simulink model "single_port_bram_test"  (R2018a)
(part 2 of 56)

      mask prompts: io_names "Names [msb...lsb]"; io_widths "Bitwidths [msb...lsb]"; io_bps "Binary pts [msb...lsb]"; io_types "Data types [msb...lsb], ufix=0, fix=1, bool=2"; show_format "Print format string?"; snap_storage "Storage medium"; snap_dram_dimm "DRAM dimm"; snap_dram_clock "DRAM clock rate"; snap_nsamples "Number of Samples (2^?)"; snap_data_width "Data width"; snap_offset "Start delay support"; snap_circap "Circular capture support"; snap_value "Extra value capture support"; snap_ext_arm "External arm support"; snap_ext_circ "External circular capture support"; snap_provide_outputs "Provide outputs"; snap_use_dsp48 "Use DSP48s to implement counters"; snap_delay "Pre-snapshot delay"; extra_names "Names [msb...lsb]"; extra_widths "Widths [msb...lsb]"; extra_bps "Binary pts [msb...lsb]"; extra_types "Data types [msb...lsb], ufix=0, fix=1, bool=2"
      mask help:
      | A wrapped snapshot block. Allows specification of inputs to a snapblock word so the toolflow can automatically set up the scope.
      | See documentation for snapshot for explanation of parameters.
      mask init:
      | bitsnap_init(gcb);
      settings: AttributesFormatString=|
      | snap(5):uf8.0,uf8.0,b,b,b = 19 bits\n32 wide, 8192 deep
      | debugID: 63192898
      mask TypeOptions snap_storage: bram | dram
      mask Callback snap_storage: bitsnap_callback();
      mask TypeOptions snap_dram_dimm: 1 | 2 | 3 | 4
      mask TypeOptions snap_dram_clock: 200 | 250 | 266 | 300 | 333
      mask TypeOptions snap_data_width: 8 | 16 | 32 | 64 | 128
      mask Callback snap_value: bitsnap_callback();
      mask Callback snap_ext_arm: bitsnap_callback();
      mask Callback snap_ext_circ: bitsnap_callback();
      mask Callback snap_provide_outputs: bitsnap_callback();
      mask DialogControl ParameterTabVar0 Prompt: Inputs
      mask DialogControl ParameterTabVar01 Prompt: Snapshot
      mask DialogControl ParameterTabVar012 Prompt: Extra Value
  snap_cnt5 : Subsystem  Tag=casper:bitsnap  Commented=on  AncestorBlock=casper_library_scopes/bitfield_snapshot  mask(bitsnap){io_names=bram_in bram_out dv_in dv_out trig], io_widths=[8 8 1 1 1], io_bps=[0 0 0 0 0], io_types=[0 0 2 2 2], show_format=on, snap_storage=bram, snap_dram_dimm=2, snap_dram_clock=250, snap_nsamples=13, snap_data_width=32, snap_offset=off, snap_circap=off, snap_value=off, snap_ext_arm=off, snap_ext_circ=off, snap_provide_outputs=on, snap_use_dsp48=on, snap_delay=2, extra_names=[c d], extra_widths=[30 2], extra_bps=[0 0], extra_types=[0 0]}
      mask prompts: io_names "Names [msb...lsb]"; io_widths "Bitwidths [msb...lsb]"; io_bps "Binary pts [msb...lsb]"; io_types "Data types [msb...lsb], ufix=0, fix=1, bool=2"; show_format "Print format string?"; snap_storage "Storage medium"; snap_dram_dimm "DRAM dimm"; snap_dram_clock "DRAM clock rate"; snap_nsamples "Number of Samples (2^?)"; snap_data_width "Data width"; snap_offset "Start delay support"; snap_circap "Circular capture support"; snap_value "Extra value capture support"; snap_ext_arm "External arm support"; snap_ext_circ "External circular capture support"; snap_provide_outputs "Provide outputs"; snap_use_dsp48 "Use DSP48s to implement counters"; snap_delay "Pre-snapshot delay"; extra_names "Names [msb...lsb]"; extra_widths "Widths [msb...lsb]"; extra_bps "Binary pts [msb...lsb]"; extra_types "Data types [msb...lsb], ufix=0, fix=1, bool=2"
      mask help:
      | A wrapped snapshot block. Allows specification of inputs to a snapblock word so the toolflow can automatically set up the scope.
      | See documentation for snapshot for explanation of parameters.
      mask init:
      | bitsnap_init(gcb);
      settings: AttributesFormatString=|
      | snap(5):uf8.0,uf8.0,b,b,b = 19 bits\n32 wide, 8192 deep
      | debugID: 63222689
      mask TypeOptions snap_storage: bram | dram
      mask Callback snap_storage: bitsnap_callback();
      mask TypeOptions snap_dram_dimm: 1 | 2 | 3 | 4
      mask TypeOptions snap_dram_clock: 200 | 250 | 266 | 300 | 333
      mask TypeOptions snap_data_width: 8 | 16 | 32 | 64 | 128
      mask Callback snap_value: bitsnap_callback();
      mask Callback snap_ext_arm: bitsnap_callback();
      mask Callback snap_ext_circ: bitsnap_callback();
      mask Callback snap_provide_outputs: bitsnap_callback();
      mask DialogControl ParameterTabVar0 Prompt: Inputs
      mask DialogControl ParameterTabVar01 Prompt: Snapshot
      mask DialogControl ParameterTabVar012 Prompt: Extra Value
  snap_cnt6 : Subsystem  Tag=casper:bitsnap  Commented=on  AncestorBlock=casper_library_scopes/bitfield_snapshot  mask(bitsnap){io_names=bram_in bram_out dv_in dv_out trig], io_widths=[8 8 1 1 1], io_bps=[0 0 0 0 0], io_types=[0 0 2 2 2], show_format=on, snap_storage=bram, snap_dram_dimm=2, snap_dram_clock=250, snap_nsamples=13, snap_data_width=32, snap_offset=off, snap_circap=off, snap_value=off, snap_ext_arm=off, snap_ext_circ=off, snap_provide_outputs=on, snap_use_dsp48=on, snap_delay=2, extra_names=[c d], extra_widths=[30 2], extra_bps=[0 0], extra_types=[0 0]}
      mask prompts: io_names "Names [msb...lsb]"; io_widths "Bitwidths [msb...lsb]"; io_bps "Binary pts [msb...lsb]"; io_types "Data types [msb...lsb], ufix=0, fix=1, bool=2"; show_format "Print format string?"; snap_storage "Storage medium"; snap_dram_dimm "DRAM dimm"; snap_dram_clock "DRAM clock rate"; snap_nsamples "Number of Samples (2^?)"; snap_data_width "Data width"; snap_offset "Start delay support"; snap_circap "Circular capture support"; snap_value "Extra value capture support"; snap_ext_arm "External arm support"; snap_ext_circ "External circular capture support"; snap_provide_outputs "Provide outputs"; snap_use_dsp48 "Use DSP48s to implement counters"; snap_delay "Pre-snapshot delay"; extra_names "Names [msb...lsb]"; extra_widths "Widths [msb...lsb]"; extra_bps "Binary pts [msb...lsb]"; extra_types "Data types [msb...lsb], ufix=0, fix=1, bool=2"
      mask help:
      | A wrapped snapshot block. Allows specification of inputs to a snapblock word so the toolflow can automatically set up the scope.
      | See documentation for snapshot for explanation of parameters.
      mask init:
      | bitsnap_init(gcb);
      settings: AttributesFormatString=|
      | snap(5):uf8.0,uf8.0,b,b,b = 19 bits\n32 wide, 8192 deep
      | debugID: 63252480
      mask TypeOptions snap_storage: bram | dram
      mask Callback snap_storage: bitsnap_callback();
      mask TypeOptions snap_dram_dimm: 1 | 2 | 3 | 4
      mask TypeOptions snap_dram_clock: 200 | 250 | 266 | 300 | 333
      mask TypeOptions snap_data_width: 8 | 16 | 32 | 64 | 128
      mask Callback snap_value: bitsnap_callback();
      mask Callback snap_ext_arm: bitsnap_callback();
      mask Callback snap_ext_circ: bitsnap_callback();
      mask Callback snap_provide_outputs: bitsnap_callback();
      mask DialogControl ParameterTabVar0 Prompt: Inputs
      mask DialogControl ParameterTabVar01 Prompt: Snapshot
      mask DialogControl ParameterTabVar012 Prompt: Extra Value
  snap_cnt7 : Subsystem  Tag=casper:bitsnap  Commented=on  AncestorBlock=casper_library_scopes/bitfield_snapshot  mask(bitsnap){io_names=bram_in bram_out dv_in dv_out trig], io_widths=[8 8 1 1 1], io_bps=[0 0 0 0 0], io_types=[0 0 2 2 2], show_format=on, snap_storage=bram, snap_dram_dimm=2, snap_dram_clock=250, snap_nsamples=13, snap_data_width=32, snap_offset=off, snap_circap=off, snap_value=off, snap_ext_arm=off, snap_ext_circ=off, snap_provide_outputs=on, snap_use_dsp48=on, snap_delay=2, extra_names=[c d], extra_widths=[30 2], extra_bps=[0 0], extra_types=[0 0]}
      mask prompts: io_names "Names [msb...lsb]"; io_widths "Bitwidths [msb...lsb]"; io_bps "Binary pts [msb...lsb]"; io_types "Data types [msb...lsb], ufix=0, fix=1, bool=2"; show_format "Print format string?"; snap_storage "Storage medium"; snap_dram_dimm "DRAM dimm"; snap_dram_clock "DRAM clock rate"; snap_nsamples "Number of Samples (2^?)"; snap_data_width "Data width"; snap_offset "Start delay support"; snap_circap "Circular capture support"; snap_value "Extra value capture support"; snap_ext_arm "External arm support"; snap_ext_circ "External circular capture support"; snap_provide_outputs "Provide outputs"; snap_use_dsp48 "Use DSP48s to implement counters"; snap_delay "Pre-snapshot delay"; extra_names "Names [msb...lsb]"; extra_widths "Widths [msb...lsb]"; extra_bps "Binary pts [msb...lsb]"; extra_types "Data types [msb...lsb], ufix=0, fix=1, bool=2"
      mask help:
      | A wrapped snapshot block. Allows specification of inputs to a snapblock word so the toolflow can automatically set up the scope.
      | See documentation for snapshot for explanation of parameters.
      mask init:
      | bitsnap_init(gcb);
      settings: AttributesFormatString=|
      | snap(5):uf8.0,uf8.0,b,b,b = 19 bits\n32 wide, 8192 deep
      | debugID: 63282271
      mask TypeOptions snap_storage: bram | dram
      mask Callback snap_storage: bitsnap_callback();
      mask TypeOptions snap_dram_dimm: 1 | 2 | 3 | 4
      mask TypeOptions snap_dram_clock: 200 | 250 | 266 | 300 | 333
      mask TypeOptions snap_data_width: 8 | 16 | 32 | 64 | 128
      mask Callback snap_value: bitsnap_callback();
      mask Callback snap_ext_arm: bitsnap_callback();
      mask Callback snap_ext_circ: bitsnap_callback();
      mask Callback snap_provide_outputs: bitsnap_callback();
      mask DialogControl ParameterTabVar0 Prompt: Inputs
      mask DialogControl ParameterTabVar01 Prompt: Snapshot
      mask DialogControl ParameterTabVar012 Prompt: Extra Value
  snap_dp1 : Subsystem  Tag=casper:bitsnap  Commented=on  AncestorBlock=casper_library_scopes/bitfield_snapshot  mask(bitsnap){io_names=bram_in bram_out dv_in dv_out trig], io_widths=[8 8 1 1 1], io_bps=[0 0 0 0 0], io_types=[0 0 2 2 2], show_format=on, snap_storage=bram, snap_dram_dimm=2, snap_dram_clock=250, snap_nsamples=13, snap_data_width=32, snap_offset=off, snap_circap=off, snap_value=off, snap_ext_arm=off, snap_ext_circ=off, snap_provide_outputs=on, snap_use_dsp48=on, snap_delay=2, extra_names=[c d], extra_widths=[30 2], extra_bps=[0 0], extra_types=[0 0]}
      mask prompts: io_names "Names [msb...lsb]"; io_widths "Bitwidths [msb...lsb]"; io_bps "Binary pts [msb...lsb]"; io_types "Data types [msb...lsb], ufix=0, fix=1, bool=2"; show_format "Print format string?"; snap_storage "Storage medium"; snap_dram_dimm "DRAM dimm"; snap_dram_clock "DRAM clock rate"; snap_nsamples "Number of Samples (2^?)"; snap_data_width "Data width"; snap_offset "Start delay support"; snap_circap "Circular capture support"; snap_value "Extra value capture support"; snap_ext_arm "External arm support"; snap_ext_circ "External circular capture support"; snap_provide_outputs "Provide outputs"; snap_use_dsp48 "Use DSP48s to implement counters"; snap_delay "Pre-snapshot delay"; extra_names "Names [msb...lsb]"; extra_widths "Widths [msb...lsb]"; extra_bps "Binary pts [msb...lsb]"; extra_types "Data types [msb...lsb], ufix=0, fix=1, bool=2"
      mask help:
      | A wrapped snapshot block. Allows specification of inputs to a snapblock word so the toolflow can automatically set up the scope.
      | See documentation for snapshot for explanation of parameters.
      mask init:
      | bitsnap_init(gcb);
      settings: AttributesFormatString=|
      | snap(5):uf8.0,uf8.0,b,b,b = 19 bits\n32 wide, 8192 deep
      | debugID: 34845580
      mask TypeOptions snap_storage: bram | dram
      mask Callback snap_storage: bitsnap_callback();
      mask TypeOptions snap_dram_dimm: 1 | 2 | 3 | 4
      mask TypeOptions snap_dram_clock: 200 | 250 | 266 | 300 | 333
      mask TypeOptions snap_data_width: 8 | 16 | 32 | 64 | 128
      mask Callback snap_value: bitsnap_callback();
      mask Callback snap_ext_arm: bitsnap_callback();
      mask Callback snap_ext_circ: bitsnap_callback();
      mask Callback snap_provide_outputs: bitsnap_callback();
      mask DialogControl ParameterTabVar0 Prompt: Inputs
      mask DialogControl ParameterTabVar01 Prompt: Snapshot
      mask DialogControl ParameterTabVar012 Prompt: Extra Value
  snap_dp2 : Subsystem  Tag=casper:bitsnap  Commented=on  AncestorBlock=casper_library_scopes/bitfield_snapshot  mask(bitsnap){io_names=bram_in bram_out dv_in dv_out trig], io_widths=[8 8 1 1 1], io_bps=[0 0 0 0 0], io_types=[0 0 2 2 2], show_format=on, snap_storage=bram, snap_dram_dimm=2, snap_dram_clock=250, snap_nsamples=13, snap_data_width=32, snap_offset=off, snap_circap=off, snap_value=off, snap_ext_arm=off, snap_ext_circ=off, snap_provide_outputs=on, snap_use_dsp48=on, snap_delay=2, extra_names=[c d], extra_widths=[30 2], extra_bps=[0 0], extra_types=[0 0]}
      mask prompts: io_names "Names [msb...lsb]"; io_widths "Bitwidths [msb...lsb]"; io_bps "Binary pts [msb...lsb]"; io_types "Data types [msb...lsb], ufix=0, fix=1, bool=2"; show_format "Print format string?"; snap_storage "Storage medium"; snap_dram_dimm "DRAM dimm"; snap_dram_clock "DRAM clock rate"; snap_nsamples "Number of Samples (2^?)"; snap_data_width "Data width"; snap_offset "Start delay support"; snap_circap "Circular capture support"; snap_value "Extra value capture support"; snap_ext_arm "External arm support"; snap_ext_circ "External circular capture support"; snap_provide_outputs "Provide outputs"; snap_use_dsp48 "Use DSP48s to implement counters"; snap_delay "Pre-snapshot delay"; extra_names "Names [msb...lsb]"; extra_widths "Widths [msb...lsb]"; extra_bps "Binary pts [msb...lsb]"; extra_types "Data types [msb...lsb], ufix=0, fix=1, bool=2"
      mask help:
      | A wrapped snapshot block. Allows specification of inputs to a snapblock word so the toolflow can automatically set up the scope.
      | See documentation for snapshot for explanation of parameters.
      mask init:
      | bitsnap_init(gcb);
      settings: AttributesFormatString=|
      | snap(5):uf8.0,uf8.0,b,b,b = 19 bits\n32 wide, 8192 deep
      | debugID: 34875371
      mask TypeOptions snap_storage: bram | dram
      mask Callback snap_storage: bitsnap_callback();
      mask TypeOptions snap_dram_dimm: 1 | 2 | 3 | 4
      mask TypeOptions snap_dram_clock: 200 | 250 | 266 | 300 | 333
      mask TypeOptions snap_data_width: 8 | 16 | 32 | 64 | 128
      mask Callback snap_value: bitsnap_callback();
      mask Callback snap_ext_arm: bitsnap_callback();
      mask Callback snap_ext_circ: bitsnap_callback();
      mask Callback snap_provide_outputs: bitsnap_callback();
      mask DialogControl ParameterTabVar0 Prompt: Inputs
      mask DialogControl ParameterTabVar01 Prompt: Snapshot
      mask DialogControl ParameterTabVar012 Prompt: Extra Value
  snap_dp3 : Subsystem  Tag=casper:bitsnap  Commented=on  AncestorBlock=casper_library_scopes/bitfield_snapshot  mask(bitsnap){io_names=bram_in bram_out dv_in dv_out trig], io_widths=[8 8 1 1 1], io_bps=[0 0 0 0 0], io_types=[0 0 2 2 2], show_format=on, snap_storage=bram, snap_dram_dimm=2, snap_dram_clock=250, snap_nsamples=13, snap_data_width=32, snap_offset=off, snap_circap=off, snap_value=off, snap_ext_arm=off, snap_ext_circ=off, snap_provide_outputs=on, snap_use_dsp48=on, snap_delay=2, extra_names=[c d], extra_widths=[30 2], extra_bps=[0 0], extra_types=[0 0]}
      mask prompts: io_names "Names [msb...lsb]"; io_widths "Bitwidths [msb...lsb]"; io_bps "Binary pts [msb...lsb]"; io_types "Data types [msb...lsb], ufix=0, fix=1, bool=2"; show_format "Print format string?"; snap_storage "Storage medium"; snap_dram_dimm "DRAM dimm"; snap_dram_clock "DRAM clock rate"; snap_nsamples "Number of Samples (2^?)"; snap_data_width "Data width"; snap_offset "Start delay support"; snap_circap "Circular capture support"; snap_value "Extra value capture support"; snap_ext_arm "External arm support"; snap_ext_circ "External circular capture support"; snap_provide_outputs "Provide outputs"; snap_use_dsp48 "Use DSP48s to implement counters"; snap_delay "Pre-snapshot delay"; extra_names "Names [msb...lsb]"; extra_widths "Widths [msb...lsb]"; extra_bps "Binary pts [msb...lsb]"; extra_types "Data types [msb...lsb], ufix=0, fix=1, bool=2"
      mask help:
      | A wrapped snapshot block. Allows specification of inputs to a snapblock word so the toolflow can automatically set up the scope.
      | See documentation for snapshot for explanation of parameters.
      mask init:
      | bitsnap_init(gcb);
      settings: AttributesFormatString=|
      | snap(5):uf8.0,uf8.0,b,b,b = 19 bits\n32 wide, 8192 deep
      | debugID: 34905162
      mask TypeOptions snap_storage: bram | dram
      mask Callback snap_storage: bitsnap_callback();
      mask TypeOptions snap_dram_dimm: 1 | 2 | 3 | 4
      mask TypeOptions snap_dram_clock: 200 | 250 | 266 | 300 | 333
      mask TypeOptions snap_data_width: 8 | 16 | 32 | 64 | 128
      mask Callback snap_value: bitsnap_callback();
      mask Callback snap_ext_arm: bitsnap_callback();
      mask Callback snap_ext_circ: bitsnap_callback();
      mask Callback snap_provide_outputs: bitsnap_callback();
      mask DialogControl ParameterTabVar0 Prompt: Inputs
      mask DialogControl ParameterTabVar01 Prompt: Snapshot
      mask DialogControl ParameterTabVar012 Prompt: Extra Value
  snap_dp4 : Subsystem  Tag=casper:bitsnap  Commented=on  AncestorBlock=casper_library_scopes/bitfield_snapshot  mask(bitsnap){io_names=bram_in bram_out dv_in dv_out trig], io_widths=[8 8 1 1 1], io_bps=[0 0 0 0 0], io_types=[0 0 2 2 2], show_format=on, snap_storage=bram, snap_dram_dimm=2, snap_dram_clock=250, snap_nsamples=13, snap_data_width=32, snap_offset=off, snap_circap=off, snap_value=off, snap_ext_arm=off, snap_ext_circ=off, snap_provide_outputs=on, snap_use_dsp48=on, snap_delay=2, extra_names=[c d], extra_widths=[30 2], extra_bps=[0 0], extra_types=[0 0]}
      mask prompts: io_names "Names [msb...lsb]"; io_widths "Bitwidths [msb...lsb]"; io_bps "Binary pts [msb...lsb]"; io_types "Data types [msb...lsb], ufix=0, fix=1, bool=2"; show_format "Print format string?"; snap_storage "Storage medium"; snap_dram_dimm "DRAM dimm"; snap_dram_clock "DRAM clock rate"; snap_nsamples "Number of Samples (2^?)"; snap_data_width "Data width"; snap_offset "Start delay support"; snap_circap "Circular capture support"; snap_value "Extra value capture support"; snap_ext_arm "External arm support"; snap_ext_circ "External circular capture support"; snap_provide_outputs "Provide outputs"; snap_use_dsp48 "Use DSP48s to implement counters"; snap_delay "Pre-snapshot delay"; extra_names "Names [msb...lsb]"; extra_widths "Widths [msb...lsb]"; extra_bps "Binary pts [msb...lsb]"; extra_types "Data types [msb...lsb], ufix=0, fix=1, bool=2"
      mask help:
      | A wrapped snapshot block. Allows specification of inputs to a snapblock word so the toolflow can automatically set up the scope.
      | See documentation for snapshot for explanation of parameters.
      mask init:
      | bitsnap_init(gcb);
      settings: AttributesFormatString=|
      | snap(5):uf8.0,uf8.0,b,b,b = 19 bits\n32 wide, 8192 deep
      | debugID: 34934953
      mask TypeOptions snap_storage: bram | dram
      mask Callback snap_storage: bitsnap_callback();
      mask TypeOptions snap_dram_dimm: 1 | 2 | 3 | 4
      mask TypeOptions snap_dram_clock: 200 | 250 | 266 | 300 | 333
      mask TypeOptions snap_data_width: 8 | 16 | 32 | 64 | 128
      mask Callback snap_value: bitsnap_callback();
      mask Callback snap_ext_arm: bitsnap_callback();
      mask Callback snap_ext_circ: bitsnap_callback();
      mask Callback snap_provide_outputs: bitsnap_callback();
      mask DialogControl ParameterTabVar0 Prompt: Inputs
      mask DialogControl ParameterTabVar01 Prompt: Snapshot
      mask DialogControl ParameterTabVar012 Prompt: Extra Value
  snap_dp5 : Subsystem  Tag=casper:bitsnap  Commented=on  AncestorBlock=casper_library_scopes/bitfield_snapshot  mask(bitsnap){io_names=bram_in bram_out dv_in dv_out trig], io_widths=[8 8 1 1 1], io_bps=[0 0 0 0 0], io_types=[0 0 2 2 2], show_format=on, snap_storage=bram, snap_dram_dimm=2, snap_dram_clock=250, snap_nsamples=13, snap_data_width=32, snap_offset=off, snap_circap=off, snap_value=off, snap_ext_arm=off, snap_ext_circ=off, snap_provide_outputs=on, snap_use_dsp48=on, snap_delay=2, extra_names=[c d], extra_widths=[30 2], extra_bps=[0 0], extra_types=[0 0]}
      mask prompts: io_names "Names [msb...lsb]"; io_widths "Bitwidths [msb...lsb]"; io_bps "Binary pts [msb...lsb]"; io_types "Data types [msb...lsb], ufix=0, fix=1, bool=2"; show_format "Print format string?"; snap_storage "Storage medium"; snap_dram_dimm "DRAM dimm"; snap_dram_clock "DRAM clock rate"; snap_nsamples "Number of Samples (2^?)"; snap_data_width "Data width"; snap_offset "Start delay support"; snap_circap "Circular capture support"; snap_value "Extra value capture support"; snap_ext_arm "External arm support"; snap_ext_circ "External circular capture support"; snap_provide_outputs "Provide outputs"; snap_use_dsp48 "Use DSP48s to implement counters"; snap_delay "Pre-snapshot delay"; extra_names "Names [msb...lsb]"; extra_widths "Widths [msb...lsb]"; extra_bps "Binary pts [msb...lsb]"; extra_types "Data types [msb...lsb], ufix=0, fix=1, bool=2"
      mask help:
      | A wrapped snapshot block. Allows specification of inputs to a snapblock word so the toolflow can automatically set up the scope.
      | See documentation for snapshot for explanation of parameters.
      mask init:
      | bitsnap_init(gcb);
      settings: AttributesFormatString=|
      | snap(5):uf8.0,uf8.0,b,b,b = 19 bits\n32 wide, 8192 deep
      | debugID: 34964744
      mask TypeOptions snap_storage: bram | dram
      mask Callback snap_storage: bitsnap_callback();
      mask TypeOptions snap_dram_dimm: 1 | 2 | 3 | 4
      mask TypeOptions snap_dram_clock: 200 | 250 | 266 | 300 | 333
      mask TypeOptions snap_data_width: 8 | 16 | 32 | 64 | 128
      mask Callback snap_value: bitsnap_callback();
      mask Callback snap_ext_arm: bitsnap_callback();
      mask Callback snap_ext_circ: bitsnap_callback();
      mask Callback snap_provide_outputs: bitsnap_callback();
      mask DialogControl ParameterTabVar0 Prompt: Inputs
      mask DialogControl ParameterTabVar01 Prompt: Snapshot
      mask DialogControl ParameterTabVar012 Prompt: Extra Value
  snap_dp6 : Subsystem  Tag=casper:bitsnap  Commented=on  AncestorBlock=casper_library_scopes/bitfield_snapshot  mask(bitsnap){io_names=bram_in bram_out dv_in dv_out trig], io_widths=[8 8 1 1 1], io_bps=[0 0 0 0 0], io_types=[0 0 2 2 2], show_format=on, snap_storage=bram, snap_dram_dimm=2, snap_dram_clock=250, snap_nsamples=13, snap_data_width=32, snap_offset=off, snap_circap=off, snap_value=off, snap_ext_arm=off, snap_ext_circ=off, snap_provide_outputs=on, snap_use_dsp48=on, snap_delay=2, extra_names=[c d], extra_widths=[30 2], extra_bps=[0 0], extra_types=[0 0]}
      mask prompts: io_names "Names [msb...lsb]"; io_widths "Bitwidths [msb...lsb]"; io_bps "Binary pts [msb...lsb]"; io_types "Data types [msb...lsb], ufix=0, fix=1, bool=2"; show_format "Print format string?"; snap_storage "Storage medium"; snap_dram_dimm "DRAM dimm"; snap_dram_clock "DRAM clock rate"; snap_nsamples "Number of Samples (2^?)"; snap_data_width "Data width"; snap_offset "Start delay support"; snap_circap "Circular capture support"; snap_value "Extra value capture support"; snap_ext_arm "External arm support"; snap_ext_circ "External circular capture support"; snap_provide_outputs "Provide outputs"; snap_use_dsp48 "Use DSP48s to implement counters"; snap_delay "Pre-snapshot delay"; extra_names "Names [msb...lsb]"; extra_widths "Widths [msb...lsb]"; extra_bps "Binary pts [msb...lsb]"; extra_types "Data types [msb...lsb], ufix=0, fix=1, bool=2"
      mask help:
      | A wrapped snapshot block. Allows specification of inputs to a snapblock word so the toolflow can automatically set up the scope.
      | See documentation for snapshot for explanation of parameters.
      mask init:
      | bitsnap_init(gcb);
      settings: AttributesFormatString=|
      | snap(5):uf8.0,uf8.0,b,b,b = 19 bits\n32 wide, 8192 deep
      | debugID: 34994535
      mask TypeOptions snap_storage: bram | dram
      mask Callback snap_storage: bitsnap_callback();
      mask TypeOptions snap_dram_dimm: 1 | 2 | 3 | 4
      mask TypeOptions snap_dram_clock: 200 | 250 | 266 | 300 | 333
      mask TypeOptions snap_data_width: 8 | 16 | 32 | 64 | 128
      mask Callback snap_value: bitsnap_callback();
      mask Callback snap_ext_arm: bitsnap_callback();
      mask Callback snap_ext_circ: bitsnap_callback();
      mask Callback snap_provide_outputs: bitsnap_callback();
      mask DialogControl ParameterTabVar0 Prompt: Inputs
      mask DialogControl ParameterTabVar01 Prompt: Snapshot
      mask DialogControl ParameterTabVar012 Prompt: Extra Value
  snap_dp7 : Subsystem  Tag=casper:bitsnap  Commented=on  AncestorBlock=casper_library_scopes/bitfield_snapshot  mask(bitsnap){io_names=bram_in bram_out dv_in dv_out trig], io_widths=[8 8 1 1 1], io_bps=[0 0 0 0 0], io_types=[0 0 2 2 2], show_format=on, snap_storage=bram, snap_dram_dimm=2, snap_dram_clock=250, snap_nsamples=13, snap_data_width=32, snap_offset=off, snap_circap=off, snap_value=off, snap_ext_arm=off, snap_ext_circ=off, snap_provide_outputs=on, snap_use_dsp48=on, snap_delay=2, extra_names=[c d], extra_widths=[30 2], extra_bps=[0 0], extra_types=[0 0]}
      mask prompts: io_names "Names [msb...lsb]"; io_widths "Bitwidths [msb...lsb]"; io_bps "Binary pts [msb...lsb]"; io_types "Data types [msb...lsb], ufix=0, fix=1, bool=2"; show_format "Print format string?"; snap_storage "Storage medium"; snap_dram_dimm "DRAM dimm"; snap_dram_clock "DRAM clock rate"; snap_nsamples "Number of Samples (2^?)"; snap_data_width "Data width"; snap_offset "Start delay support"; snap_circap "Circular capture support"; snap_value "Extra value capture support"; snap_ext_arm "External arm support"; snap_ext_circ "External circular capture support"; snap_provide_outputs "Provide outputs"; snap_use_dsp48 "Use DSP48s to implement counters"; snap_delay "Pre-snapshot delay"; extra_names "Names [msb...lsb]"; extra_widths "Widths [msb...lsb]"; extra_bps "Binary pts [msb...lsb]"; extra_types "Data types [msb...lsb], ufix=0, fix=1, bool=2"
      mask help:
      | A wrapped snapshot block. Allows specification of inputs to a snapblock word so the toolflow can automatically set up the scope.
      | See documentation for snapshot for explanation of parameters.
      mask init:
      | bitsnap_init(gcb);
      settings: AttributesFormatString=|
      | snap(5):uf8.0,uf8.0,b,b,b = 19 bits\n32 wide, 8192 deep
      | debugID: 35024326
      mask TypeOptions snap_storage: bram | dram
      mask Callback snap_storage: bitsnap_callback();
      mask TypeOptions snap_dram_dimm: 1 | 2 | 3 | 4
      mask TypeOptions snap_dram_clock: 200 | 250 | 266 | 300 | 333
      mask TypeOptions snap_data_width: 8 | 16 | 32 | 64 | 128
      mask Callback snap_value: bitsnap_callback();
      mask Callback snap_ext_arm: bitsnap_callback();
      mask Callback snap_ext_circ: bitsnap_callback();
      mask Callback snap_provide_outputs: bitsnap_callback();
      mask DialogControl ParameterTabVar0 Prompt: Inputs
      mask DialogControl ParameterTabVar01 Prompt: Snapshot
      mask DialogControl ParameterTabVar012 Prompt: Extra Value
  snap_dp8 : Subsystem  Tag=casper:bitsnap  Commented=on  AncestorBlock=casper_library_scopes/bitfield_snapshot  mask(bitsnap){io_names=bram_in bram_out dv_in dv_out trig], io_widths=[8 8 1 1 1], io_bps=[0 0 0 0 0], io_types=[0 0 2 2 2], show_format=on, snap_storage=bram, snap_dram_dimm=2, snap_dram_clock=250, snap_nsamples=13, snap_data_width=32, snap_offset=off, snap_circap=off, snap_value=off, snap_ext_arm=off, snap_ext_circ=off, snap_provide_outputs=on, snap_use_dsp48=on, snap_delay=2, extra_names=[c d], extra_widths=[30 2], extra_bps=[0 0], extra_types=[0 0]}
      mask prompts: io_names "Names [msb...lsb]"; io_widths "Bitwidths [msb...lsb]"; io_bps "Binary pts [msb...lsb]"; io_types "Data types [msb...lsb], ufix=0, fix=1, bool=2"; show_format "Print format string?"; snap_storage "Storage medium"; snap_dram_dimm "DRAM dimm"; snap_dram_clock "DRAM clock rate"; snap_nsamples "Number of Samples (2^?)"; snap_data_width "Data width"; snap_offset "Start delay support"; snap_circap "Circular capture support"; snap_value "Extra value capture support"; snap_ext_arm "External arm support"; snap_ext_circ "External circular capture support"; snap_provide_outputs "Provide outputs"; snap_use_dsp48 "Use DSP48s to implement counters"; snap_delay "Pre-snapshot delay"; extra_names "Names [msb...lsb]"; extra_widths "Widths [msb...lsb]"; extra_bps "Binary pts [msb...lsb]"; extra_types "Data types [msb...lsb], ufix=0, fix=1, bool=2"
      mask help:
      | A wrapped snapshot block. Allows specification of inputs to a snapblock word so the toolflow can automatically set up the scope.
      | See documentation for snapshot for explanation of parameters.
      mask init:
      | bitsnap_init(gcb);
      settings: AttributesFormatString=|
      | snap(5):uf8.0,uf8.0,b,b,b = 19 bits\n32 wide, 8192 deep
      | debugID: 35054117
      mask TypeOptions snap_storage: bram | dram
      mask Callback snap_storage: bitsnap_callback();
      mask TypeOptions snap_dram_dimm: 1 | 2 | 3 | 4
      mask TypeOptions snap_dram_clock: 200 | 250 | 266 | 300 | 333
      mask TypeOptions snap_data_width: 8 | 16 | 32 | 64 | 128
      mask Callback snap_value: bitsnap_callback();
      mask Callback snap_ext_arm: bitsnap_callback();
      mask Callback snap_ext_circ: bitsnap_callback();
      mask Callback snap_provide_outputs: bitsnap_callback();
      mask DialogControl ParameterTabVar0 Prompt: Inputs
      mask DialogControl ParameterTabVar01 Prompt: Snapshot
      mask DialogControl ParameterTabVar012 Prompt: Extra Value
  sys_rst : Subsystem  Tag=xps:sw_reg  AncestorBlock=xps_library/Memory/software_register  mask(swreg){io_dir=From Processor, io_delay=1, init_val=0, sample_period=1, names=rst, bitwidths=1, bin_pts=0, arith_types=2, sim_port=on, show_format=on}
      mask prompts: io_dir "I/O direction"; io_delay "I/O delay"; init_val "Initial Value"; sample_period "Sample period"; names "Bitfield names [msb...lsb]"; bitwidths "Bitfield widths"; bin_pts "Bitfield binary pts"; arith_types "Bitfield types, ufix=0, fix=1, bool=2"; sim_port "Provide sim input/output?"; show_format "Print format string?"
      mask help: A 32-bit software-accessible register. Can be divided into bitfields of varying widths and types using the fields in the block mask.
      mask init:
      | swreg_init(gcb)
      settings: AttributesFormatString=1input:b = 1 bits
      mask TypeOptions io_dir: To Processor | From Processor
      mask Callback io_dir:
      | mask_enables = get_param(gcb, 'MaskEnables');
      | mask_names = get_param(gcb, 'MaskNames');
      | if strcmp(get_param(gcb, 'io_dir'), 'To Processor'),
      |     mask_enables{ismember(mask_names, 'sample_period')} = 'off';
      | else
      |     mask_enables{ismember(mask_names, 'sample_period')} = 'on';
      | end
      | set_param(gcb, 'MaskEnables', mask_enables);
      mask DialogControl ParameterTabVar0 Prompt: Setup
  sys_start : Subsystem  Tag=xps:sw_reg  AncestorBlock=xps_library/Memory/software_register  mask(swreg){io_dir=From Processor, io_delay=1, init_val=0, sample_period=1, names=en, bitwidths=1, bin_pts=0, arith_types=2, sim_port=on, show_format=on}
      mask prompts: io_dir "I/O direction"; io_delay "I/O delay"; init_val "Initial Value"; sample_period "Sample period"; names "Bitfield names [msb...lsb]"; bitwidths "Bitfield widths"; bin_pts "Bitfield binary pts"; arith_types "Bitfield types, ufix=0, fix=1, bool=2"; sim_port "Provide sim input/output?"; show_format "Print format string?"
      mask help: A 32-bit software-accessible register. Can be divided into bitfields of varying widths and types using the fields in the block mask.
      mask init:
      | swreg_init(gcb)
      settings: AttributesFormatString=1input:b = 1 bits
      mask TypeOptions io_dir: To Processor | From Processor
      mask Callback io_dir:
      | mask_enables = get_param(gcb, 'MaskEnables');
      | mask_names = get_param(gcb, 'MaskNames');
      | if strcmp(get_param(gcb, 'io_dir'), 'To Processor'),
      |     mask_enables{ismember(mask_names, 'sample_period')} = 'off';
      | else
      |     mask_enables{ismember(mask_names, 'sample_period')} = 'on';
      | end
      | set_param(gcb, 'MaskEnables', mask_enables);
      mask DialogControl ParameterTabVar0 Prompt: Setup
  xsg_core_config : xps_library/Platforms/SKARAB  Tag=xps:xsg  hw_sys=SKARAB:xc7vx690t  clk_src=sys_clk  clk_rate=238  sample_period=1  synthesis_tool=XST
      settings: SourceProductName=CASPER XPS Blockset
  wires:
  ram/1 -> Gateway Out5/1, pipeline3/1(d)
  pipeline112/1(q) -> [forty_gbe_rx_eof]
  Constant23/1 -> [s256_v]
  Logical7/1 -> Logical5/1
  [board_in_fault] -> Inverter/1
  [force_gbe_txen] -> Logical7/2
  pipeline97/1(q) -> gbe0/4(tx_dest_ip)
  pipeline62/1(q) -> [forty_gbe_rx_valid]
  Logical2/1 -> gbe0/3(tx_valid)
  [s256_eof] -> Delay4/2
  pipeline114/1(q) -> [forty_gbe_rx_overrun]
  gbe0/1(led_up) -> pipeline100/1(d)
  pipeline108/1(q) -> [forty_gbe_rx_data]
  pipeline102/1(q) -> [forty_gbe_led_tx]
  Constant22/1 -> [s256_d]
  pipeline104/1(q) -> [forty_gbe_tx_of]
  pipeline22/1(q) -> gbe_status/2(out_led_rx)
  pipeline103/1(q) -> [forty_gbe_tx_full]
  Logical5/1 -> Delay4/1
  pipeline99/1(q) -> gbe0/1(rst)
  [s256_eof] -> Logical3/2
  pipeline20/1(q) -> gbe_status/1(out_led_up)
  Constant7/1 -> [force_gbe_txen], [gbe_txen]
  gbe0/3(led_tx) -> pipeline102/1(d)
  gbe0/14(rx_dest_port) -> pipeline116/1(d)
  gbe0/11(rx_bad_frame) -> pipeline113/1(d)
  [s256_v] -> Logical2/2
  Constant5/1 -> [gbe_cnt_rst]
  [forty_gbe_led_rx] -> pipeline22/1(d)
  gbe0/6(rx_data) -> pipeline108/1(d)
  Constant21/1 -> gbe0/8(rx_overrun_ack)
  pipeline100/1(q) -> [forty_gbe_led_up]
  [forty_gbe_led_up] -> pipeline20/1(d)
  [forty_gbe_led_tx] -> pipeline51/1(d)
  pipeline31/1(q) -> gbe0/9(debug_rst)
  [gbe_cnt_rst] -> pipeline31/1(d)
  gbe0/5(tx_overflow) -> pipeline104/1(d)
  Constant24/1 -> [s256_eof]
  pipeline/1(q) -> rx_dest_ip/1(out_reg)
  pipeline115/1(q) -> [rx_dest_ip]
  gbe0/12(rx_overrun) -> pipeline114/1(d)
  [gbe_rst] -> pipeline99/1(d)
  gbe0/8(rx_source_ip) -> pipeline110/1(d)
  pipeline111/1(q) -> [forty_gbe_rx_src_port]
  Constant20/1 -> gbe0/7(rx_ack)
  gbe0/9(rx_source_port) -> pipeline111/1(d)
  Constant25/1 -> [s256_port]
  gbe0/4(tx_afull) -> pipeline103/1(d)
  Constant18/1 -> [board_in_fault]
  pipeline116/1(q) -> [rx_dest_port]
  gbe0/13(rx_dest_ip) -> pipeline115/1(d)
  gbe0/10(rx_end_of_frame) -> pipeline112/1(d)
  [s256_d] -> pipeline98/1(d)
  pipeline51/1(q) -> gbe_status/3(out_led_tx)
  pipeline110/1(q) -> [forty_gbe_rx_src_ip]
  Logical3/1 -> gbe0/6(tx_end_of_frame)
  [s256_port] -> pipeline96/1(d)
  Inverter/1 -> Logical7/1
  pipeline96/1(q) -> gbe0/5(tx_dest_port)
  [rx_dest_ip] -> pipeline/1(d)
  Constant26/1 -> [s256_ip]
  pipeline113/1(q) -> [forty_gbe_rx_bad]
  [gbe_txen] -> Logical5/2
  gbe0/2(led_rx) -> pipeline101/1(d)
  Constant6/1 -> [gbe_rst]
  [s256_ip] -> pipeline97/1(d)
  pipeline98/1(q) -> gbe0/2(tx_data)
  pipeline101/1(q) -> [forty_gbe_led_rx]
  Delay4/1 -> Logical2/1, Logical3/1
  gbe0/7(rx_valid) -> pipeline62/1(d)
  Constant32/1 -> sys_rst/1(sim_1)
  sys_rst/1(in_rst) -> pipeline19/1(d)
  sys_start/1(in_en) -> pipeline1/1(d)
  Constant1/1 -> sys_start/1(sim_1)
  From/1 -> pipeline5/1(d), pipeline8/1(d), Counter1/1
  pipeline2/1(q) -> snap_cnt/1(in_bram_in)
  pipeline3/1(q) -> snap_cnt/2(in_bram_out)
  pipeline4/1(q) -> snap_cnt/6(we)
  pipeline5/1(q) -> snap_cnt/5(in_trig)
  pkt_len/1(in_len) -> pipeline28/1(d)
  Constant33/1 -> pkt_len/1(sim_1)
  Constant4/1 -> gap_len/1(sim_1)
  gap_len/1(in_offset) -> pipeline125/1(d)
  Delay/1 -> Gateway Out6/1, pipeline7/1(d)
  pipeline7/1(q) -> snap_cnt/4(in_dv_out)
  pipeline6/1(q) -> snap_cnt/3(in_dv_in)
  pipeline8/1(q) -> snap_cnt/7(trig)
  counter/1 -> ram/1
  Counter1/1 -> Gateway Out3/1, ram/2, pipeline2/1(d)
  From3/1 -> pipeline4/1(d), pipeline6/1(d), counter/1, ram/3, Gateway Out4/1, ram/4, Delay/1, Counter1/2
  Gateway Out3/1 -> To Workspace3/1
  Gateway Out4/1 -> To Workspace4/1
  Gateway Out5/1 -> To Workspace5/1
  Gateway Out6/1 -> To Workspace6/1
  Gateway Out10/1 -> To Workspace10/1
  Gateway Out9/1 -> To Workspace9/1
  Gateway Out8/1 -> To Workspace8/1
  Gateway Out7/1 -> To Workspace7/1
  From5/1 -> Counter2/2, Delay3/1, ram1/4, Gateway Out8/1, ram1/3, counter1/1, pipeline13/1(d), pipeline11/1(d)
  Counter2/1 -> pipeline9/1(d), ram1/2, Gateway Out7/1
  counter1/1 -> ram1/1
  pipeline15/1(q) -> snap_cnt1/7(trig)
  pipeline13/1(q) -> snap_cnt1/3(in_dv_in)
  pipeline14/1(q) -> snap_cnt1/4(in_dv_out)
  Delay3/1 -> pipeline14/1(d), Gateway Out10/1
  pipeline12/1(q) -> snap_cnt1/5(in_trig)
  pipeline11/1(q) -> snap_cnt1/6(we)
  pipeline10/1(q) -> snap_cnt1/2(in_bram_out)
  pipeline9/1(q) -> snap_cnt1/1(in_bram_in)
  From1/1 -> Counter2/1, pipeline15/1(d), pipeline12/1(d)
  ram1/1 -> pipeline10/1(d), Gateway Out9/1
  ram2/1 -> Gateway Out14/1, pipeline16/1(d)
  From6/1 -> pipeline18/1(d), pipeline24/1(d), Counter3/1
  pipeline25/1(q) -> snap_cnt2/1(in_bram_in)
  pipeline16/1(q) -> snap_cnt2/2(in_bram_out)
  pipeline17/1(q) -> snap_cnt2/6(we)
  pipeline18/1(q) -> snap_cnt2/5(in_trig)
  Delay5/1 -> Gateway Out11/1, pipeline23/1(d)
  pipeline23/1(q) -> snap_cnt2/4(in_dv_out)
  pipeline21/1(q) -> snap_cnt2/3(in_dv_in)
  pipeline24/1(q) -> snap_cnt2/7(trig)
  counter2/1 -> ram2/1
  Counter3/1 -> Gateway Out12/1, ram2/2, pipeline25/1(d)
  From9/1 -> pipeline17/1(d), pipeline21/1(d), counter2/1, ram2/3, Gateway Out13/1, ram2/4, Delay5/1, Counter3/2
  Gateway Out12/1 -> To Workspace12/1
  Gateway Out13/1 -> To Workspace13/1
  Gateway Out14/1 -> To Workspace14/1
  Gateway Out11/1 -> To Workspace11/1
  Gateway Out15/1 -> To Workspace15/1
  Gateway Out18/1 -> To Workspace18/1
  Gateway Out17/1 -> To Workspace17/1
  Gateway Out16/1 -> To Workspace16/1
  From11/1 -> Counter4/2, Delay6/1, ram3/4, Gateway Out17/1, ram3/3, counter3/1, pipeline30/1(d), pipeline27/1(d)
  Counter4/1 -> pipeline34/1(d), ram3/2, Gateway Out16/1
  counter3/1 -> ram3/1
  pipeline33/1(q) -> snap_cnt3/7(trig)
  pipeline30/1(q) -> snap_cnt3/3(in_dv_in)
  pipeline32/1(q) -> snap_cnt3/4(in_dv_out)
  Delay6/1 -> pipeline32/1(d), Gateway Out15/1
  pipeline29/1(q) -> snap_cnt3/5(in_trig)
  pipeline27/1(q) -> snap_cnt3/6(we)
  pipeline26/1(q) -> snap_cnt3/2(in_bram_out)
  pipeline34/1(q) -> snap_cnt3/1(in_bram_in)
  From10/1 -> Counter4/1, pipeline33/1(d), pipeline29/1(d)
  ram3/1 -> pipeline26/1(d), Gateway Out18/1
  ram4/1 -> Gateway Out22/1, pipeline35/1(d)
  From12/1 -> pipeline37/1(d), pipeline40/1(d), Counter5/1
  pipeline41/1(q) -> snap_cnt4/1(in_bram_in)
  pipeline35/1(q) -> snap_cnt4/2(in_bram_out)
  pipeline36/1(q) -> snap_cnt4/6(we)
  pipeline37/1(q) -> snap_cnt4/5(in_trig)
  Delay7/1 -> Gateway Out19/1, pipeline39/1(d)
  pipeline39/1(q) -> snap_cnt4/4(in_dv_out)
  pipeline38/1(q) -> snap_cnt4/3(in_dv_in)
  pipeline40/1(q) -> snap_cnt4/7(trig)
  counter4/1 -> ram4/1
  Counter5/1 -> Gateway Out20/1, ram4/2, pipeline41/1(d)
  From13/1 -> pipeline36/1(d), pipeline38/1(d), counter4/1, ram4/3, Gateway Out21/1, ram4/4, Delay7/1, Counter5/2
  Gateway Out20/1 -> To Workspace20/1
  Gateway Out21/1 -> To Workspace21/1
  Gateway Out22/1 -> To Workspace22/1
  Gateway Out19/1 -> To Workspace19/1
  Gateway Out23/1 -> To Workspace23/1
  Gateway Out26/1 -> To Workspace26/1
  Gateway Out25/1 -> To Workspace25/1
  Gateway Out24/1 -> To Workspace24/1
  From15/1 -> Counter6/2, Delay8/1, ram5/4, Gateway Out25/1, ram5/3, counter5/1, pipeline45/1(d), pipeline43/1(d)
  Counter6/1 -> pipeline48/1(d), ram5/2, Gateway Out24/1
  counter5/1 -> ram5/1
  pipeline47/1(q) -> snap_cnt5/7(trig)
  pipeline45/1(q) -> snap_cnt5/3(in_dv_in)
  pipeline46/1(q) -> snap_cnt5/4(in_dv_out)
  Delay8/1 -> pipeline46/1(d), Gateway Out23/1
  pipeline44/1(q) -> snap_cnt5/5(in_trig)
  pipeline43/1(q) -> snap_cnt5/6(we)
  pipeline42/1(q) -> snap_cnt5/2(in_bram_out)
  pipeline48/1(q) -> snap_cnt5/1(in_bram_in)
  From14/1 -> Counter6/1, pipeline47/1(d), pipeline44/1(d)
  ram5/1 -> pipeline42/1(d), Gateway Out26/1
  ram6/1 -> Gateway Out30/1, pipeline49/1(d)
  From18/1 -> pipeline52/1(d), pipeline55/1(d), Counter7/1
  pipeline56/1(q) -> snap_cnt6/1(in_bram_in)
  pipeline49/1(q) -> snap_cnt6/2(in_bram_out)
  pipeline50/1(q) -> snap_cnt6/6(we)
  pipeline52/1(q) -> snap_cnt6/5(in_trig)
  Delay9/1 -> Gateway Out27/1, pipeline54/1(d)
  pipeline54/1(q) -> snap_cnt6/4(in_dv_out)
  pipeline53/1(q) -> snap_cnt6/3(in_dv_in)
  pipeline55/1(q) -> snap_cnt6/7(trig)
  counter6/1 -> ram6/1
  Counter7/1 -> Gateway Out28/1, ram6/2, pipeline56/1(d)
  From19/1 -> pipeline50/1(d), pipeline53/1(d), counter6/1, ram6/3, Gateway Out29/1, ram6/4, Delay9/1, Counter7/2
  Gateway Out28/1 -> To Workspace28/1
  Gateway Out29/1 -> To Workspace29/1
  Gateway Out30/1 -> To Workspace30/1
  Gateway Out27/1 -> To Workspace27/1
  Gateway Out31/1 -> To Workspace31/1
  Gateway Out34/1 -> To Workspace34/1
  Gateway Out33/1 -> To Workspace33/1
  Gateway Out32/1 -> To Workspace32/1
  From21/1 -> Counter8/2, Delay10/1, ram7/4, Gateway Out33/1, ram7/3, counter7/1, pipeline60/1(d), pipeline58/1(d)
  Counter8/1 -> pipeline64/1(d), ram7/2, Gateway Out32/1
  counter7/1 -> ram7/1
  pipeline63/1(q) -> snap_cnt7/7(trig)
  pipeline60/1(q) -> snap_cnt7/3(in_dv_in)
  pipeline61/1(q) -> snap_cnt7/4(in_dv_out)
  Delay10/1 -> pipeline61/1(d), Gateway Out31/1
  pipeline59/1(q) -> snap_cnt7/5(in_trig)
  pipeline58/1(q) -> snap_cnt7/6(we)
  pipeline57/1(q) -> snap_cnt7/2(in_bram_out)
  pipeline64/1(q) -> snap_cnt7/1(in_bram_in)
  From20/1 -> Counter8/1, pipeline63/1(d), pipeline59/1(d)
  ram7/1 -> pipeline57/1(d), Gateway Out34/1
  From22/1 -> pipeline67/1(d), pipeline70/1(d), Counter9/1
  pipeline71/1(q) -> snap_dp3/1(in_bram_in)
  pipeline65/1(q) -> snap_dp3/2(in_bram_out)
  pipeline66/1(q) -> snap_dp3/6(we)
  pipeline67/1(q) -> snap_dp3/5(in_trig)
  pipeline69/1(q) -> snap_dp3/4(in_dv_out)
  pipeline68/1(q) -> snap_dp3/3(in_dv_in)
  pipeline70/1(q) -> snap_dp3/7(trig)
  Counter9/1 -> Dual Port RAM/2, Gateway Out81/1, pipeline71/1(d)
  counter8/1 -> Dual Port RAM/4, Dual Port RAM/1
  Constant/1 -> Dual Port RAM/6
  Constant2/1 -> Dual Port RAM/5
  Dual Port RAM/2 -> Gateway Out48/1, pipeline65/1(d)
  Delay11/1 -> Gateway Out47/1, pipeline69/1(d)
  Gateway Out44/1 -> To Workspace44/1
  Gateway Out43/1 -> To Workspace43/1
  Gateway Out42/1 -> To Workspace42/1
  Gateway Out41/1 -> To Workspace41/1
  Gateway Out40/1 -> To Workspace40/1
  Delay12/1 -> pipeline76/1(d), Gateway Out41/1
  Dual Port RAM1/2 -> pipeline72/1(d), Gateway Out40/1
  Constant8/1 -> Dual Port RAM1/5
  Constant3/1 -> Dual Port RAM1/6
  counter9/1 -> Dual Port RAM1/1, Dual Port RAM1/4, Gateway Out42/1
  From30/1 -> Dual Port RAM1/8, Gateway Out44/1, counter9/1, Dual Port RAM1/3, Dual Port RAM1/7, pipeline75/1(d), pipeline73/1(d), Delay12/1, Counter11/2
  Counter11/1 -> pipeline78/1(d), Dual Port RAM1/2, Gateway Out43/1
  pipeline77/1(q) -> snap_dp1/7(trig)
  pipeline75/1(q) -> snap_dp1/3(in_dv_in)
  pipeline76/1(q) -> snap_dp1/4(in_dv_out)
  pipeline74/1(q) -> snap_dp1/5(in_trig)
  pipeline73/1(q) -> snap_dp1/6(we)
  pipeline72/1(q) -> snap_dp1/2(in_bram_out)
  pipeline78/1(q) -> snap_dp1/1(in_bram_in)
  From26/1 -> Counter11/1, pipeline77/1(d), pipeline74/1(d)
  From33/1 -> pipeline88/1(d), pipeline91/1(d), Counter13/1
  pipeline92/1(q) -> snap_dp2/1(in_bram_in)
  pipeline86/1(q) -> snap_dp2/2(in_bram_out)
  pipeline87/1(q) -> snap_dp2/6(we)
  pipeline88/1(q) -> snap_dp2/5(in_trig)
  pipeline90/1(q) -> snap_dp2/4(in_dv_out)
  pipeline89/1(q) -> snap_dp2/3(in_dv_in)
  pipeline91/1(q) -> snap_dp2/7(trig)
  Counter13/1 -> Dual Port RAM3/2, pipeline92/1(d)
  From34/1 -> Counter13/2, Delay14/1, pipeline87/1(d), pipeline89/1(d), Dual Port RAM3/7, Dual Port RAM3/3, counter11/1, Dual Port RAM3/8
  counter11/1 -> Dual Port RAM3/4, Dual Port RAM3/1
  Constant11/1 -> Dual Port RAM3/6
  Constant12/1 -> Dual Port RAM3/5
  Dual Port RAM3/2 -> Gateway Out49/1, pipeline86/1(d)
  Delay14/1 -> Gateway Out50/1, pipeline90/1(d)
  Delay18/1 -> Gateway Out52/1, pipeline136/1(d)
  Dual Port RAM7/2 -> Gateway Out51/1, pipeline132/1(d)
  Constant16/1 -> Dual Port RAM7/5
  Constant15/1 -> Dual Port RAM7/6
  counter13/1 -> Dual Port RAM7/1, Dual Port RAM7/4
  From42/1 -> Dual Port RAM7/8, counter13/1, Dual Port RAM7/3, Dual Port RAM7/7, pipeline135/1(d), pipeline133/1(d), Delay18/1, Counter16/2
  Counter16/1 -> pipeline138/1(d), Dual Port RAM7/2
  pipeline137/1(q) -> snap_dp6/7(trig)
  pipeline135/1(q) -> snap_dp6/3(in_dv_in)
  pipeline136/1(q) -> snap_dp6/4(in_dv_out)
  pipeline134/1(q) -> snap_dp6/5(in_trig)
  pipeline133/1(q) -> snap_dp6/6(we)
  pipeline132/1(q) -> snap_dp6/2(in_bram_out)
  pipeline138/1(q) -> snap_dp6/1(in_bram_in)
  From41/1 -> Counter16/1, pipeline137/1(d), pipeline134/1(d)
  From39/1 -> pipeline127/1(d), pipeline130/1(d), Counter15/1
  pipeline131/1(q) -> snap_dp8/1(in_bram_in)
  pipeline124/1(q) -> snap_dp8/2(in_bram_out)
  pipeline126/1(q) -> snap_dp8/6(we)
  pipeline127/1(q) -> snap_dp8/5(in_trig)
  pipeline129/1(q) -> snap_dp8/4(in_dv_out)
  pipeline128/1(q) -> snap_dp8/3(in_dv_in)
  pipeline130/1(q) -> snap_dp8/7(trig)
  Counter15/1 -> Dual Port RAM6/2, pipeline131/1(d)
  From40/1 -> Counter15/2, Delay17/1, pipeline126/1(d), pipeline128/1(d), Dual Port RAM6/7, Dual Port RAM6/3, counter12/1, Dual Port RAM6/8
  counter12/1 -> Dual Port RAM6/4, Dual Port RAM6/1
  Constant28/1 -> Dual Port RAM6/6
  Constant14/1 -> Dual Port RAM6/5
  Dual Port RAM6/2 -> Gateway Out55/1, pipeline124/1(d)
  Delay17/1 -> Gateway Out56/1, pipeline129/1(d)
  From37/1 -> pipeline119/1(d), pipeline122/1(d), Counter14/1
  pipeline123/1(q) -> snap_dp5/1(in_bram_in)
  pipeline117/1(q) -> snap_dp5/2(in_bram_out)
  pipeline118/1(q) -> snap_dp5/6(we)
  pipeline119/1(q) -> snap_dp5/5(in_trig)
  pipeline121/1(q) -> snap_dp5/4(in_dv_out)
  pipeline120/1(q) -> snap_dp5/3(in_dv_in)
  pipeline122/1(q) -> snap_dp5/7(trig)
  Counter14/1 -> Gateway Out38/1, Dual Port RAM5/2, pipeline123/1(d)
  From38/1 -> Counter14/2, Delay16/1, pipeline118/1(d), pipeline120/1(d), Dual Port RAM5/7, Dual Port RAM5/3, counter15/1, Gateway Out39/1, Dual Port RAM5/8
  counter15/1 -> Gateway Out37/1, Dual Port RAM5/4, Dual Port RAM5/1
  Constant19/1 -> Dual Port RAM5/6
  Constant27/1 -> Dual Port RAM5/5
  Dual Port RAM5/2 -> Gateway Out35/1, pipeline117/1(d)
  Delay16/1 -> Gateway Out36/1, pipeline121/1(d)
  Gateway Out35/1 -> To Workspace35/1
  Gateway Out36/1 -> To Workspace36/1
  Gateway Out37/1 -> To Workspace37/1
  Gateway Out38/1 -> To Workspace38/1
  Gateway Out39/1 -> To Workspace39/1
  Delay15/1 -> Gateway Out54/1, pipeline106/1(d)
  Dual Port RAM4/2 -> Gateway Out53/1, pipeline93/1(d)
  Constant17/1 -> Dual Port RAM4/5
  Constant13/1 -> Dual Port RAM4/6
  counter14/1 -> Dual Port RAM4/1, Dual Port RAM4/4
  From36/1 -> Dual Port RAM4/8, counter14/1, Dual Port RAM4/3, Dual Port RAM4/7, pipeline105/1(d), pipeline94/1(d), Delay15/1, Counter17/2
  Counter17/1 -> pipeline109/1(d), Dual Port RAM4/2
  pipeline107/1(q) -> snap_dp7/7(trig)
  pipeline105/1(q) -> snap_dp7/3(in_dv_in)
  pipeline106/1(q) -> snap_dp7/4(in_dv_out)
  pipeline95/1(q) -> snap_dp7/5(in_trig)
  pipeline94/1(q) -> snap_dp7/6(we)
  pipeline93/1(q) -> snap_dp7/2(in_bram_out)
  pipeline109/1(q) -> snap_dp7/1(in_bram_in)
  From35/1 -> Counter17/1, pipeline107/1(d), pipeline95/1(d)
  From23/1 -> Delay11/1, pipeline66/1(d), pipeline68/1(d), Dual Port RAM/7, Dual Port RAM/8, counter8/1, Dual Port RAM/3, Counter9/2
  Gateway Out48/1 -> To Workspace48/1
  Gateway Out49/1 -> To Workspace49/1
  Gateway Out47/1 -> To Workspace47/1
  Gateway Out50/1 -> To Workspace50/1
  Gateway Out51/1 -> To Workspace51/1
  Gateway Out52/1 -> To Workspace52/1
  Gateway Out53/1 -> To Workspace53/1
  Gateway Out54/1 -> To Workspace54/1
  Gateway Out55/1 -> To Workspace55/1
  Gateway Out56/1 -> To Workspace56/1
  Delay28/1 -> Gateway Out62/1, pipeline165/1(d)
  Delay29/1 -> Delay24/1
  Delay24/1 -> Delay28/1
  From53/1 -> pipeline162/1(d), pipeline164/1(d), ram11/4, Delay19/2, Delay23/2, ram11/3, Delay29/1, counter19/1, Counter21/2
  Gateway Out69/1 -> To Workspace69/1
  Gateway Out68/1 -> To Workspace68/1
  Gateway Out62/1 -> To Workspace62/1
  Gateway Out57/1 -> To Workspace57/1
  Delay23/1 -> pipeline161/1(d), Gateway Out57/1
  Delay19/1 -> Delay23/1
  ram11/1 -> Delay19/1
  From52/1 -> pipeline163/1(d), pipeline166/1(d), Counter21/1
  pipeline160/1(q) -> snap_cnt11/1(in_bram_in)
  pipeline161/1(q) -> snap_cnt11/2(in_bram_out)
  pipeline162/1(q) -> snap_cnt11/6(we)
  pipeline163/1(q) -> snap_cnt11/5(in_trig)
  pipeline165/1(q) -> snap_cnt11/4(in_dv_out)
  pipeline164/1(q) -> snap_cnt11/3(in_dv_in)
  pipeline166/1(q) -> snap_cnt11/7(trig)
  counter19/1 -> ram11/1, Gateway Out68/1
  Counter21/1 -> Gateway Out69/1, ram11/2, pipeline160/1(d)
  Delay35/1 -> pipeline172/1(d), Gateway Out74/1
  Gateway Out74/1 -> To Workspace74/1
  Delay34/1 -> Delay35/1
  From55/1 -> Counter22/2, Delay33/2, Gateway Out71/1, ram12/4, ram12/3, Delay34/1, counter20/1, pipeline171/1(d), pipeline169/1(d)
  Counter22/1 -> pipeline167/1(d), ram12/2, Gateway Out73/1
  counter20/1 -> Gateway Out72/1, ram12/1
  pipeline173/1(q) -> snap_cnt12/7(trig)
  pipeline171/1(q) -> snap_cnt12/3(in_dv_in)
  pipeline172/1(q) -> snap_cnt12/4(in_dv_out)
  pipeline170/1(q) -> snap_cnt12/5(in_trig)
  pipeline169/1(q) -> snap_cnt12/6(we)
  pipeline168/1(q) -> snap_cnt12/2(in_bram_out)
  pipeline167/1(q) -> snap_cnt12/1(in_bram_in)
  From54/1 -> Counter22/1, pipeline173/1(d), pipeline170/1(d)
  ram12/1 -> Delay33/1
  Delay33/1 -> Gateway Out70/1, pipeline168/1(d)
  Gateway Out70/1 -> To Workspace70/1
  Gateway Out71/1 -> To Workspace71/1
  Gateway Out72/1 -> To Workspace72/1
  Gateway Out73/1 -> To Workspace73/1
  Gateway Out81/1 -> To Workspace81/1
  Gateway Out82/1 -> To Workspace82/1
  Gateway Out45/1 -> To Workspace45/1
  Gateway Out46/1 -> To Workspace46/1
  From32/1 -> Counter12/2, Dual Port RAM2/3, counter10/1, Dual Port RAM2/8, Dual Port RAM2/7, pipeline82/1(d), pipeline80/1(d), Delay13/1
  Delay13/1 -> pipeline83/1(d), Gateway Out45/1
  Dual Port RAM2/2 -> pipeline79/1(d), Gateway Out46/1
  Constant10/1 -> Dual Port RAM2/5
  Constant9/1 -> Dual Port RAM2/6
  counter10/1 -> Dual Port RAM2/4, Dual Port RAM2/1
  Counter12/1 -> pipeline85/1(d), Gateway Out82/1, Dual Port RAM2/2
  pipeline84/1(q) -> snap_dp4/7(trig)
  pipeline82/1(q) -> snap_dp4/3(in_dv_in)
  pipeline83/1(q) -> snap_dp4/4(in_dv_out)
  pipeline81/1(q) -> snap_dp4/5(in_trig)
  pipeline80/1(q) -> snap_dp4/6(we)
  pipeline79/1(q) -> snap_dp4/2(in_bram_out)
  pipeline85/1(q) -> snap_dp4/1(in_bram_in)
  From31/1 -> Counter12/1, pipeline84/1(d), pipeline81/1(d)
  gap_scale/1(in_len) -> pipeline140/1(d)
  Constant31/1 -> gap_scale/1(sim_1)
  gap_sel/1(in_sel) -> pipeline141/1(d)
  Constant34/1 -> gap_sel/1(sim_1)
  Constant29/1 -> pkt_scale/1(sim_1)
  pkt_scale/1(in_len) -> pipeline139/1(d)
  Constant37/1 -> pkt_sel/1(sim_1)
  pkt_sel/1(in_sel) -> pipeline142/1(d)
  pipeline19/1(q) -> Subsystem/1(rst)
  pipeline1/1(q) -> Subsystem/2(start)
  pipeline141/1(q) -> Subsystem/3(gap_sel)
  pipeline125/1(q) -> Subsystem/4(gap_len)
  pipeline140/1(q) -> Subsystem/5(gap_scale)
  pipeline142/1(q) -> Subsystem/6(pkt_sel)
  pipeline28/1(q) -> Subsystem/7(pkt_length)
  pipeline139/1(q) -> Subsystem/8(pkt_len_scale)
  Subsystem/1(Sync Out) -> [sync_gen]
  Subsystem/2(DV out) -> [dv_gen]
